simulink model "Apps2_Model"  (R2019a)
settings: Solver=VariableStepAuto  StartTime=0.0  StopTime=10.0  RelTol=1e-3
PostLoadFcn:
  | AppsInit
StopFcn:
  | AppsVisualize
settings Model: Creator=G5  LastModifiedBy=G5
settings DataIOCC: LoadExternalInput=on  SaveFormat=Array

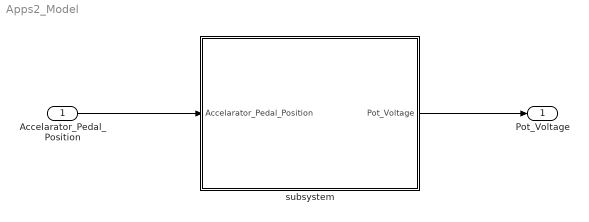
== system Apps2_Model ==
  Accelarator_Pedal_Position : Inport
  subsystem : Subsystem
      mask help: Apps
  Pot_Voltage : Outport
  wires:
  Accelarator_Pedal_Position/1 -> subsystem/1(Accelarator_Pedal_Position)
  subsystem/1(Pot_Voltage) -> Pot_Voltage/1

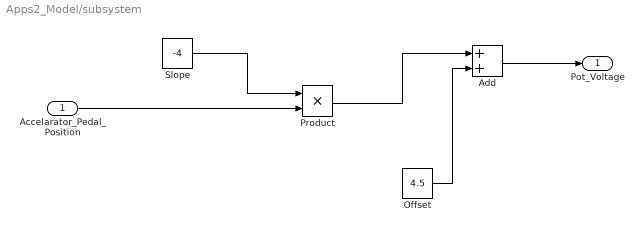
== system Apps2_Model/subsystem ==
  Accelarator_Pedal_Position : Inport
  Add : Sum
  Offset : Constant  Value=4.5
  Product : Product
  Slope : Constant  Value=-4
  Pot_Voltage : Outport
  wires:
  Slope/1 -> Product/1
  Accelarator_Pedal_Position/1 -> Product/2
  Product/1 -> Add/1
  Offset/1 -> Add/2
  Add/1 -> Pot_Voltage/1
